simulink model "gm_hdlconvert_tb"  (R2017a)
settings: Solver=VariableStepAuto  StartTime=0.0  StopTime=3* 2^8  RelTol=1e-3  EnableMultiTasking=on
libraries: lib_dsphdltypes_v1 x6, dspsrcs4 x1
settings Model: Creator=babstm  LastModifiedBy=mbabst
settings DataIOCC: LimitDataPoints=on
settings OptimizationCC: BlockReduction=off  ConditionallyExecuteInputs=off  DefaultParameterBehavior=Inlined  LifeSpan=inf
settings DebuggingCC: AlgebraicLoopMsg=error  InheritedTsInSrcMsg=none  AllowSymbolicDim=off  SFUnexpectedBacktrackingDiag=warning  SFNoUnconditionalDefaultTransitionDiag=warning  SFExecutionAtInitializationDiag=none
settings HardwareCC: ProdBitPerPointer=32  ProdBitPerSizeT=32  ProdBitPerPtrDiffT=32  ProdLargestAtomicFloat=None  ProdIntDivRoundTo=Undefined  ProdEndianess=Unspecified  ProdWordSize=32  ProdHWDeviceType=ASIC/FPGA->ASIC/FPGA  ProdEqTarget=off
settings ModelReferenceCC: PropagateSignalLabelsOutOfModel=off
settings GRTTargetCC: TargetLangStandard=C89/C90 (ANSI)
settings ConfigComp: CovMetricSettings=dw  CovHtmlReporting=on  CovSaveCumulativeToWorkspaceVar=on  CovSaveSingleToWorkspaceVar=on  CovExternalEMLEnable=off

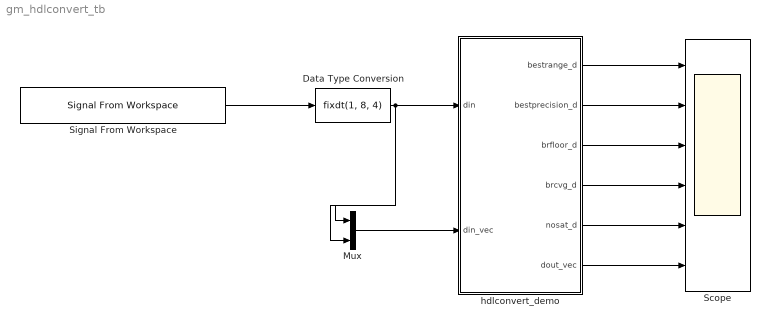
== system gm_hdlconvert_tb ==
  Data Type Conversion : DataTypeConversion  OutDataTypeStr=fixdt(1, 8, 4)  ConvertRealWorld=Stored Integer (SI)
  Mux : Mux  Inputs=2
  Scope : Scope  NumInputPorts=6
  Signal From Workspace : dspsrcs4/Signal From Workspace  X=[(0:2^7-1) (2^7-1-2:-1:-2^7 ) (-2^7 : -1) ]  Ts=1  nsamps=1  OutputAfterFinalValue=Cyclic repetition  ignoreOrWarnInputAndFrameLengths=on  OutputFrames=off
  hdlconvert_demo : Subsystem
  wires:
  hdlconvert_demo/6(dout_vec) -> Scope/6
  hdlconvert_demo/5(nosat_d) -> Scope/5
  hdlconvert_demo/4(brcvg_d) -> Scope/4
  hdlconvert_demo/3(brfloor_d) -> Scope/3
  hdlconvert_demo/2(bestprecision_d) -> Scope/2
  hdlconvert_demo/1(bestrange_d) -> Scope/1
  Mux/1 -> hdlconvert_demo/2(din_vec)
  Data Type Conversion/1 -> hdlconvert_demo/1(din), Mux/1, Mux/2
  Signal From Workspace/1 -> Data Type Conversion/1

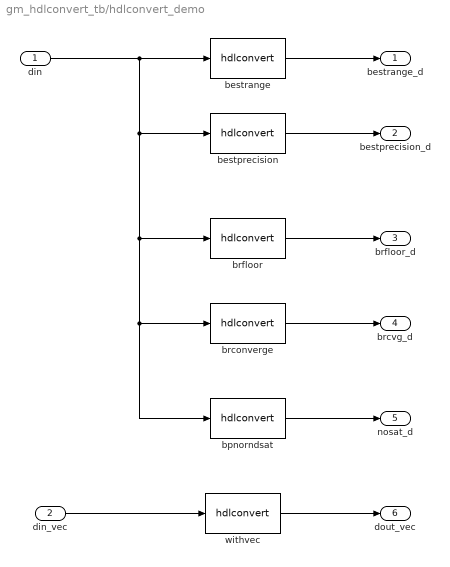
== system gm_hdlconvert_tb/hdlconvert_demo ==
  din : Inport
  din_vec : Inport  Port=2
  bestprecision : lib_dsphdltypes_v1/hdlconvert  signed=Inherit  maxwidth=6  extend=on  scaleopt=Best Precision  Sforce=0  roundMode=Nearest  saturate=on
      settings: SourceProductName=DSPHDL Library
  bestrange : lib_dsphdltypes_v1/hdlconvert  signed=Inherit  maxwidth=6  extend=on  scaleopt=Best Range  Sforce=0  roundMode=Nearest  saturate=on
      settings: SourceProductName=DSPHDL Library
  bpnorndsat : lib_dsphdltypes_v1/hdlconvert  signed=Inherit  maxwidth=6  extend=on  scaleopt=Best Precision  Sforce=0  roundMode=Floor  saturate=off
      settings: SourceProductName=DSPHDL Library
  brconverge : lib_dsphdltypes_v1/hdlconvert  signed=Inherit  maxwidth=6  extend=on  scaleopt=Best Range  Sforce=0  roundMode=Convergent  saturate=on
      settings: SourceProductName=DSPHDL Library
  brfloor : lib_dsphdltypes_v1/hdlconvert  signed=Inherit  maxwidth=6  extend=on  scaleopt=Best Range  Sforce=0  roundMode=Floor  saturate=on
      settings: SourceProductName=DSPHDL Library
  withvec : lib_dsphdltypes_v1/hdlconvert  signed=Inherit  maxwidth=6  extend=on  scaleopt=Best Precision  Sforce=0  roundMode=Floor  saturate=off
      settings: SourceProductName=DSPHDL Library
  bestrange_d : Outport
  bestprecision_d : Outport  Port=2
  brfloor_d : Outport  Port=3
  brcvg_d : Outport  Port=4
  nosat_d : Outport  Port=5
  dout_vec : Outport  Port=6
  wires:
  bpnorndsat/1 -> nosat_d/1
  brconverge/1 -> brcvg_d/1
  brfloor/1 -> brfloor_d/1
  bestprecision/1 -> bestprecision_d/1
  withvec/1 -> dout_vec/1
  din_vec/1 -> withvec/1
  bestrange/1 -> bestrange_d/1
  din/1 -> bestprecision/1, brconverge/1, bpnorndsat/1, brfloor/1, bestrange/1
